simulink model "PP2_Q2"  (Simulink 7.9)
settings: Solver=ode45  StartTime=0.0  StopTime=350  RelTol=1e-3
values from neighbouring files (symbols this model uses):
  BetaZero = 1/N    (= 2.5e-06)    [PP2_Q2_prog.m]
  Eta = 2.5    [PP2_Q2_prog.m]
  Gamma = 0.025    [PP2_Q2_prog.m]
  IZero = 2    [PP2_Q2_prog.m]
  Mu = 0.08/N    (= 2e-07)    [PP2_Q2_prog.m]
  N = 400000    [PP2_Q2_prog.m]
settings Model: Creator=Basundhara  LastModifiedBy=Basundhara

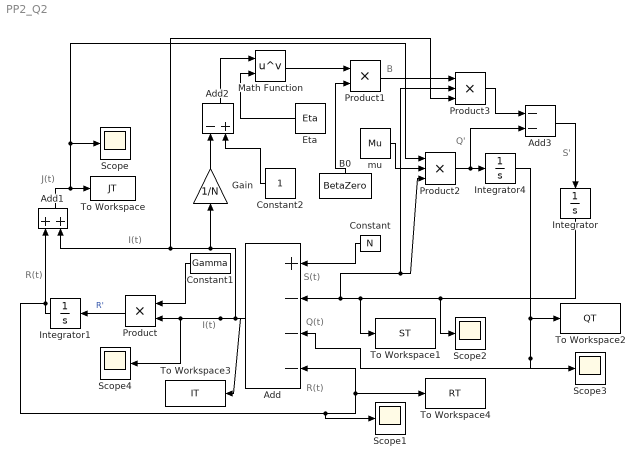
== system PP2_Q2 ==
  note: S(t)
  note: I(t)
  note: Q(t)
  note: R(t)
  note: I(t)
  note: J(t)
  note: Q'
  note: B
  note: S'
  note: R(t)
  Add : Sum  Inputs=+---
  Add1 : Sum
  Add2 : Sum  Inputs=-+
  Add3 : Sum  Inputs=--
  B0 : Constant  Value=BetaZero
  Constant : Constant  Value=N
  Constant1 : Constant  Value=Gamma
  Constant2 : Constant
  Eta : Constant  Value=Eta
  Gain : Gain  Gain=1/N
  Integrator : Integrator  InitialCondition=N-IZero
  Integrator1 : Integrator
  Integrator4 : Integrator
  Math Function : Math  Operator=pow  SaturateOnIntegerOverflow=on
  Product : Product  RndMeth=Zero
  Product1 : Product  RndMeth=Zero
  Product2 : Product  Inputs=3  RndMeth=Zero
  Product3 : Product  Inputs=3  RndMeth=Zero
  Scope{,1..4} (5 alike) : Scope
      Scope2 settings: SaveName=ScopeData2
      Scope3 settings: SaveName=ScopeData3
      Scope4 settings: SaveName=ScopeData4
  To Workspace : ToWorkspace  VariableName=JT  SampleTime=-1  SaveFormat=Structure With Time
  To Workspace1 : ToWorkspace  VariableName=ST  SampleTime=-1  SaveFormat=Structure With Time
  To Workspace2 : ToWorkspace  VariableName=QT  SampleTime=-1  SaveFormat=Structure With Time
  To Workspace3 : ToWorkspace  VariableName=IT  SampleTime=-1  SaveFormat=Structure With Time
  To Workspace4 : ToWorkspace  VariableName=RT  SampleTime=-1  SaveFormat=Structure With Time
  mu : Constant  Value=Mu
  wires:
  Integrator/1 -> Add/2, Product2/3, Product3/2, To Workspace1/1, Scope2/1
  Constant/1 -> Add/1
  Constant1/1 -> Product/1
  Add/1 -> Gain/1, Add1/2, Product3/3, To Workspace3/1, Product/2, Scope4/1
  Product/1 -> Integrator1/1  "R'"
  Integrator1/1 -> Add1/1, To Workspace4/1, Add/4, Scope1/1
  Add1/1 -> To Workspace/1, Product2/1, Scope/1
  Gain/1 -> Add2/1
  Constant2/1 -> Add2/2
  Add2/1 -> Math Function/1
  Eta/1 -> Math Function/2
  Math Function/1 -> Product1/1
  B0/1 -> Product1/2
  mu/1 -> Product2/2
  Product2/1 -> Integrator4/1, Add3/2
  Integrator4/1 -> To Workspace2/1, Scope3/1, Add/3
  Product1/1 -> Product3/1
  Product3/1 -> Add3/1
  Add3/1 -> Integrator/1
